simulink model "theta_double"  (R2019a)
settings: Solver=VariableStepAuto  StartTime=0.0  StopTime=10.0  MaxStep=1e-3  RelTol=1e-3
values from neighbouring files (symbols this model uses):
  g = 9.8    [bakr_theta.m]
  l = values(i)    [bakr_theta.m]
settings Model: Creator=LEGION  LastModifiedBy=LEGION

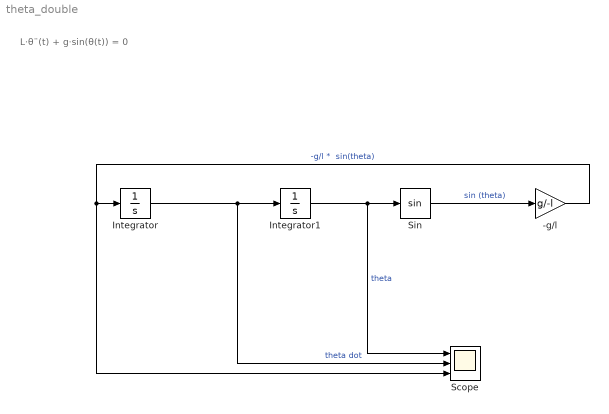
== system theta_double ==
  note: L⋅θ¨(t) + g⋅sin(θ(t)) = 0
  "-g/l " : Gain  Gain=g/-l
  Integrator : Integrator  InitialCondition=1
  Integrator1 : Integrator  InitialCondition=1
  Scope : Scope  NumInputPorts=3
  Sin : Trigonometry
  wires:
  Integrator/1 -> Scope/2, Integrator1/1  "theta dot"
  Integrator1/1 -> Scope/1, Sin/1  "theta"
  Sin/1 -> "-g/l "/1  "sin (theta)"
  "-g/l "/1 -> Scope/3, Integrator/1  "-g/l *  sin(theta)"
